simulink model "DCMotor"  (R2020a)
settings: Solver=VariableStepAuto  StartTime=0.0  StopTime=10.0  RelTol=1e-3
values from neighbouring files (symbols this model uses):
  b = input('Enter the value for Friction Torque B= ')    [Ajith007ElectroMechanicalSys.m]
  J = 0.01    [EX10.m]    (also in Untitled.m)
  K = input('Enter the value of Spring constant K=')    [Ajith007MechanicalSys.m]    (also in BodePlot.m = 5; EX10 (1).m = input('Enter Spring Constant: '); Ex81.m = input("Enter the value of gain for required steady state err; Exercise_6.m = 1)
  L = input('Enter the value for inductance L=')    [ElecSys2nd.m]    (also in Untitled.m = 0.5)
  R = input('Enter resistance R=')    [Ajith007ElectricalSys.m]    (also in ElecSys1st.m = input('Enter the value for resistance R= '); ElecSys2nd.m = input('Enter the value for resistance R= '); Untitled.m = 1)
settings Model: Creator=Harini Prakash  LastModifiedBy=Harini Prakash

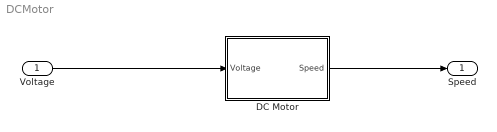
== system DCMotor ==
  Voltage : Inport
  DC Motor : Subsystem
  Speed : Outport
  wires:
  Voltage/1 -> DC Motor/1(Voltage)
  DC Motor/1(Speed) -> Speed/1

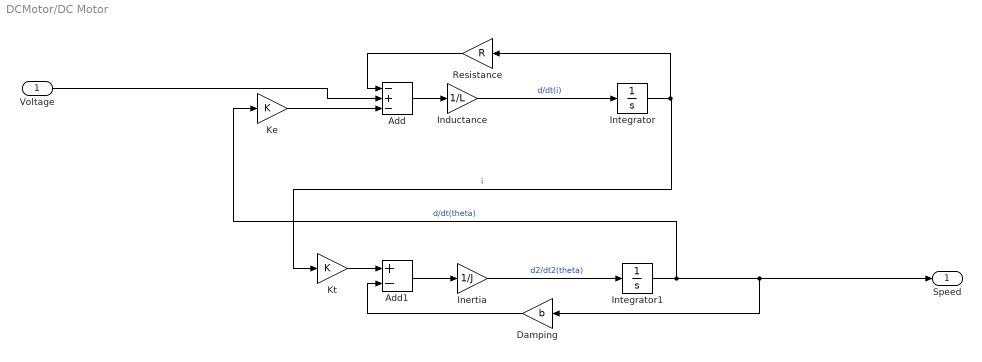
== system DCMotor/DC Motor ==
  Voltage : Inport
  Add : Sum  Inputs=-+-
  Add1 : Sum  Inputs=+-
  Damping : Gain  Gain=b
  Inductance : Gain  Gain=1/L
  Inertia : Gain  Gain=1/J
  Integrator : Integrator
  Integrator1 : Integrator
  Ke : Gain  Gain=K
  Kt : Gain  Gain=K
  Resistance : Gain  Gain=R
  Speed : Outport
  wires:
  Inductance/1 -> Integrator/1  "d/dt(i)"
  Kt/1 -> Add1/1
  Voltage/1 -> Add/2
  Integrator1/1 -> Speed/1, Damping/1, Ke/1  "d/dt(theta)"
  Inertia/1 -> Integrator1/1  "d2/dt2(theta)"
  Add/1 -> Inductance/1
  Add1/1 -> Inertia/1
  Resistance/1 -> Add/1
  Ke/1 -> Add/3
  Integrator/1 -> Resistance/1, Kt/1  "i"
  Damping/1 -> Add1/2
